simulink model "SubsystemAtomic"  (R2024a)
settings: Solver=FixedStepDiscrete  StartTime=0.0  StopTime=10.0  FixedStep=1  RelTol=1e-3  EnableMultiTasking=on
undefined symbols (not defined in the file): DiscIntNeverNeededParam
libraries: CodeGenerationWidgets x2
Description:
  | Preserving Subsystem Boundaries in Generated Code
  | 
  | This model shows how to preserve the boundary of a virtual subsystem
  | in the generated code.
settings Model: Creator=The MathWorks, Inc.  LastModifiedBy=The MathWorks, Inc.
settings SolverCC: AlgebraicLoopSolver=TrustRegion
settings DataIOCC: LimitDataPoints=on  SaveFormat=Array  SaveOutput=off  SaveTime=off  ReturnWorkspaceOutputs=off  SignalLoggingName=sigsOut
settings OptimizationCC: DefaultParameterBehavior=Inlined  InlineInvariantSignals=on  ExpressionDepthLimit=2147483647  StateBitsets=on  DataBitsets=on  EfficientFloat2IntCast=on  EfficientMapNaN2IntZero=off  LifeSpan=inf
settings DebuggingCC: MergeDetectMultiDrivingBlocksExec=none  CheckExecutionContextPreStartOutputMsg=on  FcnCallInpInsideContextMsg=warning  UnconnectedInputMsg=warning  UnconnectedOutputMsg=warning  UnconnectedLineMsg=warning  AllowSymbolicDim=off  StateNameClashWarn=warning  SubsystemReferenceDiagnosticForUnitTest=warning  StrictBusMsg=ErrorOnBusTreatedAsVector  SymbolicDimsDataTypeCodeGenerationDiagnostic=none  SFUnexpectedBacktrackingDiag=warning  SFNoUnconditionalDefaultTransitionDiag=warning  SFExecutionAtInitializationDiag=none  ArithmeticOperatorsInVariantConditions=warning
settings HardwareCC: TargetHWDeviceType=Generic->32-bit Embedded Processor
settings ModelReferenceCC: EnableRefExpFcnMdlSchedulingChecks=on  PropagateSignalLabelsOutOfModel=off
settings SFSimCC: SimUseLocalCustomCode=off
settings RTWCC: TLCOptions=-p0 -aWarnNonSaturatedBlocks=0  GenerateReport=on  RTWVerbose=off  RTWUseLocalCustomCode=off  LaunchReport=on  GPUComputeCapability=3.5
settings CodeAppCC: ForceParamTrailComments=on  StateflowObjectComments=on
settings GRTTargetCC: TargetFcnLib=ansi_tfl_tmw.mat  TargetLangStandard=C89/C90 (ANSI)  UtilityFuncGeneration=Shared location  MatFileLogging=off
settings ConfigComp: CovMetricSettings=dw  CovSaveCumulativeToWorkspaceVar=on  CovSaveSingleToWorkspaceVar=on  CovExternalEMLEnable=off

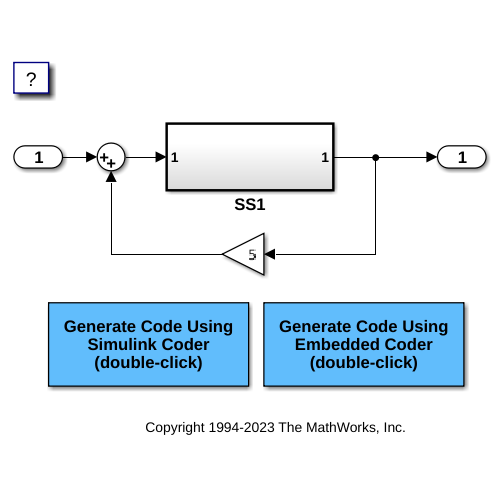
[thumbnail: Simulink's stored preview of the top-level diagram]
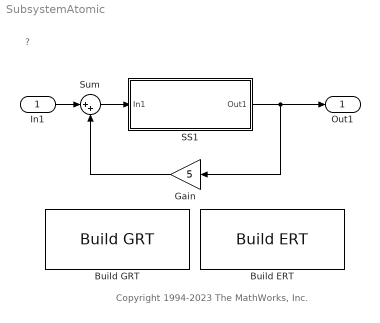
== system SubsystemAtomic ==
  note: Copyright 1994-2023 The MathWorks, Inc.
  note: ?
  In1 : Inport  OutDataTypeStr=double  PortDimensions=1  SampleTime=1
  Build ERT : CodeGenerationWidgets/Build ERT  attrib_overrides={}
  Build GRT : CodeGenerationWidgets/Build GRT  attrib_overrides={}
  Gain : Gain  Gain=5  SaturateOnIntegerOverflow=on  OutDataTypeStr=Inherit: Same as input  ParamDataTypeStr=Inherit: Same as input
  SS1 : Subsystem  TreatAsAtomicUnit=on  RTWFcnName=myfun  RTWFileName=myfile
      settings: RTWFcnNameOpts=User specified
  Sum : Sum  Inputs=|++
  Out1 : Outport  VectorParamsAs1DForOutWhenUnconnected=off
  wires:
  Sum/1 -> SS1/1(In1)
  In1/1 -> Sum/1
  SS1/1(Out1) -> Out1/1, Gain/1
  Gain/1 -> Sum/2

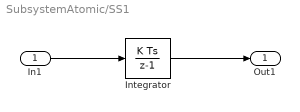
== system SubsystemAtomic/SS1 ==
  In1 : Inport
  Integrator : DiscreteIntegrator  ICPrevOutput=DiscIntNeverNeededParam  ICPrevScaledInput=DiscIntNeverNeededParam
  Out1 : Outport  VectorParamsAs1DForOutWhenUnconnected=off
  wires:
  In1/1 -> Integrator/1
  Integrator/1 -> Out1/1
